simulink model "data_analysis"  (Simulink 7.6)
settings: Solver=FixedStepDiscrete  StartTime=0.0  StopTime=0  RelTol=1e-3
undefined symbols (not defined in the file or in its folder): jet
libraries: vipsnks x1, viptextngfix x1, vipsrcs x1, viptransforms x1
settings Model: Creator=auvt  LastModifiedBy=auvt
settings OptimizationCC: OptimizeModelRefInitCode=on  LifeSpan=1
settings RTWCC: SystemTargetFile=ert.tlc  GenCodeOnly=on  TemplateMakefile=ert_default_tmf  Description=Real-Time Workshop Embedded Coder  GenerateReport=on  ProcessScript=ert_make_rtw_hook  IncludeHyperlinkInReport=on  LaunchReport=on
settings CodeAppCC: IgnoreCustomStorageClasses=off
settings ERTTargetCC: MultiwordLength=2048  GenerateSampleERTMain=on  ERTCustomFileTemplate=example_file_process.tlc  ConvertIfToSwitch=off

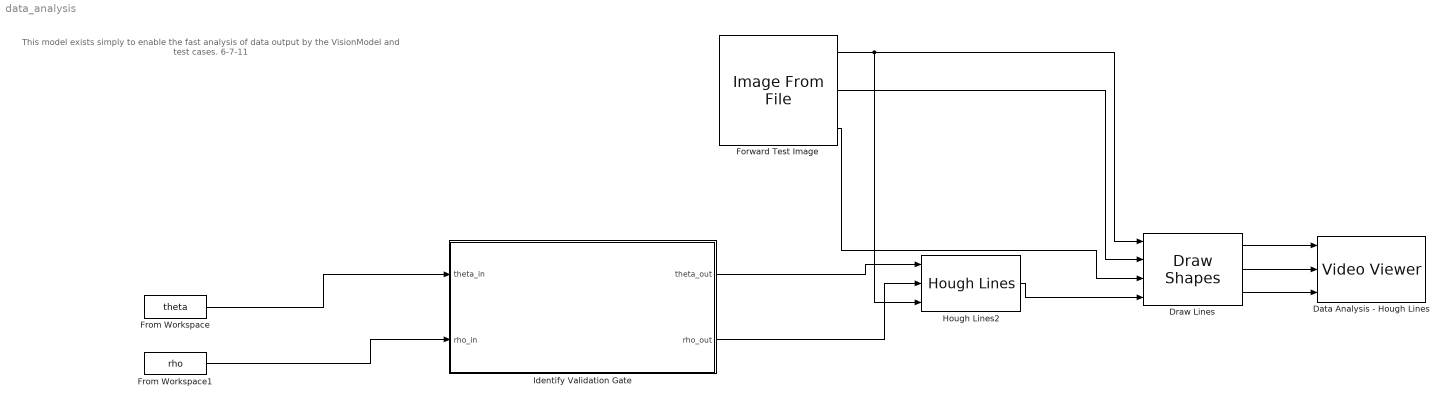
== system data_analysis ==
  note: This model exists simply to enable
      | the fast analysis of data output
      | by the VisionModel and test cases.
      |
      | 6-7-11
  Data Analysis - Hough Lines : vipsnks/Video Viewer  DialogControllerArgs=DataTag1  inputType=Obsolete7b  imagePorts=Separate color signals  useColorMap=off  colormapValue=jet(256)  specRange=off  minInputVal=0  maxInputVal=255  FigPos=[1001 849 410 300]  AxisZoom=on  trueSizedOnce=off  OpenAtMdlStart=on
  Draw Lines : viptextngfix/Draw Shapes  DialogController=vipDDGCreate  DialogControllerArgs=DataTag2  shape=Lines  fill=off  fillClrSource=Specify via dialog  display=User-specified value  intensity=200  color=[.8 .8 .8]  opacity=0.6  viewport=Entire image  antialiasing=off  inType=Obsolete  imagePorts=Separate color signals  prodOutputMode=Binary point scaling  prodOutputWordLength=32  prodOutputFracLength=14  memoryMode=Specify word length  memoryWordLength=16  memoryFracLength=15  roundingMode=Floor  overflowMode=off
  Forward Test Image : vipsrcs/Image From File  Tag=vipblks_nd  DialogController=vipDDGCreate  DialogControllerArgs=DataTag3  SystemSampleTime=-1  FileName=/home/auvt/auvc/src/vision/Modified_Files_for_Testing/Images/gate9.PNG  imagePorts=Separate color signals  Ts=-1  ImageDataType=double  Signed=on  WordLength=16  sdImageDataType=uint(8)  FractionLengthMode=User-defined  FractionLength=15  OutPortLabels=R|G|B
  From Workspace : FromWorkspace  VariableName=theta  SampleTime=0
  From Workspace1 : FromWorkspace  VariableName=rho  SampleTime=0
  Hough Lines2 : viptransforms/Hough Lines  DialogController=vipDDGCreate  DialogControllerArgs=DataTag4  sineCompMethod=Trigonometric function  thetaRes=pi/180  firstCoeffMode=Specify word length  firstCoeffWordLength=16  firstCoeffFracLength=15  prodOutputMode=Binary point scaling  prodOutputWordLength=32  prodOutputFracLength=16  roundingMode=Nearest  overflowMode=on
  Identify Validation Gate : Stateflow chart  TreatAsAtomicUnit=on  SystemSampleTime=[1/30 0]
  wires:
  From Workspace/1 -> Identify Validation Gate/1(theta_in)
  From Workspace1/1 -> Identify Validation Gate/2(rho_in)
  Identify Validation Gate/1(theta_out) -> Hough Lines2/1
  Identify Validation Gate/2(rho_out) -> Hough Lines2/2
  Hough Lines2/1 -> Draw Lines/4
  Forward Test Image/1 -> Draw Lines/1, Hough Lines2/3
  Forward Test Image/2 -> Draw Lines/2
  Forward Test Image/3 -> Draw Lines/3
  Draw Lines/1 -> Data Analysis - Hough Lines/1
  Draw Lines/2 -> Data Analysis - Hough Lines/2
  Draw Lines/3 -> Data Analysis - Hough Lines/3

== matlab function Identify Validation Gate ==
  data: theta_in input double; rho_in input double; theta_out output double; rho_out output double
function [theta_out, rho_out] = chooseHoughLines(theta_in, rho_in)
%#eml

nmax = 150;


theta_out = zeros(1, nmax);
rho_out = zeros(1, nmax);

eps_theta = 8*pi/180;



for i = 1:nmax-1
    
    condition1 = ( abs(theta_in(i) - pi/2) <= eps_theta || abs(theta_in(i) + pi/2) <= eps_theta );
    condition2 = ( abs(theta_in(i) - 0) <= eps_theta );
    if( condition1 || condition2 )
        theta_out(i) = theta_in(i);
        rho_out(i) = rho_in(i);
    end
end

return
